simulink model "Day02"  (R2024b)
settings: Solver=VariableStepAuto  StartTime=0.0  StopTime=10.0  RelTol=1e-3
settings Model: Creator=jun_mac  LastModifiedBy=jun_mac

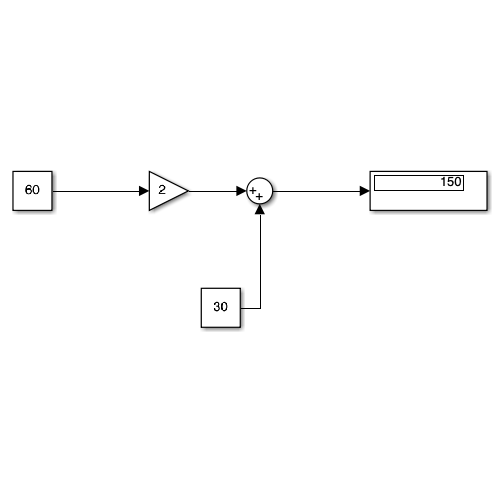
[thumbnail: Simulink's stored preview of the top-level diagram]
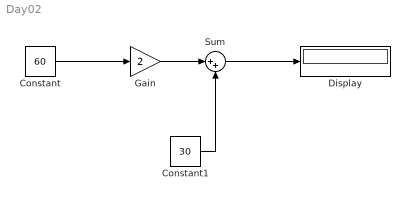
== system Day02 ==
  Constant : Constant  Value=60
  Constant1 : Constant  Value=30
  Display : Display
  Gain : Gain  Gain=2
  Sum : Sum  Inputs=|++
  wires:
  Constant/1 -> Gain/1
  Sum/1 -> Display/1
  Constant1/1 -> Sum/2
  Gain/1 -> Sum/1
